simulink model "ss512"  (Simulink 8.1)
settings: Solver=ode45  StartTime=0.0  StopTime=50  FixedStep=T  RelTol=1e-3
values from neighbouring files (symbols this model uses):
  A = [0 1; 0 0]    [ss1_init.m]    (also in ss512_init.m = [0 0 1 0; ss51_init.m = [0 0 1 0)
  B = [0; 1]    [ss1_init.m]    (also in ss512_init.m = [0; 0; 0; 1]; ss51_init.m = [0; 0; 0; 1])
  C = eye(2)    [ss1_init.m]    (also in ss512_init.m = eye(n); ss51_init.m = eye(n))
  D = [0; 0]    [ss1_init.m]    (also in ss512_init.m = zeros([n 1]); ss51_init.m = zeros([n 1]))
  H = [1 0]    [ex8_init.m]    (also in ss512_init.m = [1 0 0 0])
  K1 = myacker(Phi, Gamma, z1)    [ss512_init.m]    (also in ss51_init.m)
  K2 = myacker(Phi, Gamma, z2)    [ss512_init.m]    (also in ss51_init.m)
  Lp = acker(Phi', H', p)'    [ex8_init.m]    (also in ss512_init.m = acker(Phi', H', z3)')
  Phi = [1 T; 0 1]    [ex8_init.m]
  T = 0.1    [ex8_init.m]    (also in ss1_init.m; ss512_init.m = 0.4; ss51_init.m = 0.4)
  x1 = [1; 0]    [ex8_init.m]    (also in ss1_init.m = [1; 1]; ss512_init.m = [1; 0; 0; 0]; ss51_init.m = [1; 0; 0; 0])
undefined symbols (not defined in the file or in its folder): Gamma
settings Model: Creator=jmahler  LastModifiedBy=jmahler
settings DataIOCC: SignalLoggingSaveFormat=Dataset
settings OptimizationCC: ExpressionDepthLimit=128
settings DebuggingCC: FcnCallInpInsideContextMsg=EnableAllAsError
settings GRTTargetCC: CombineOutputUpdateFcns=on  GRTInterface=off

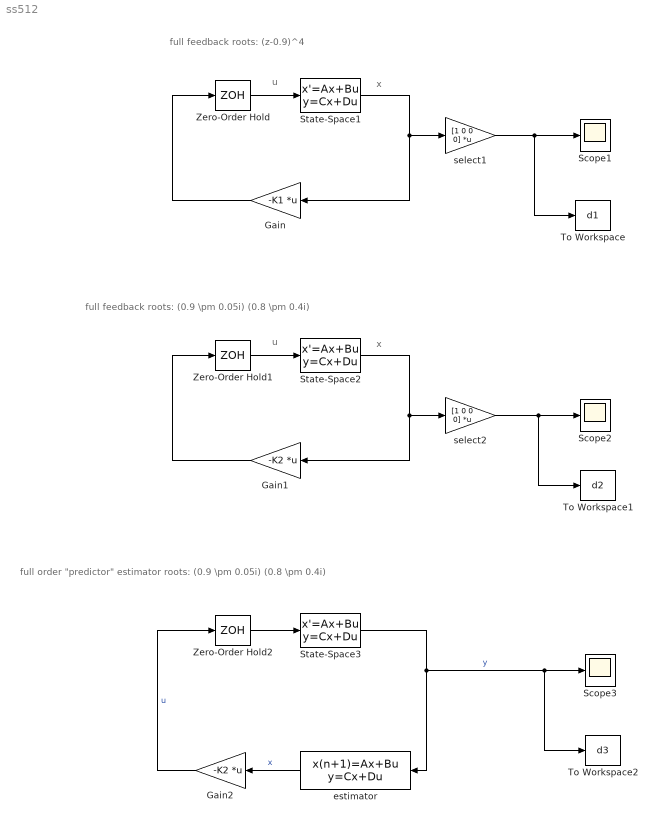
== system ss512 ==
  note: full feedback
      | roots: (z-0.9)^4
  note: u
  note: x
  note: u
  note: x
  note: full feedback
      | roots: (0.9 \pm 0.05i) (0.8 \pm 0.4i)
  note: full order "predictor" estimator
      | roots: (0.9 \pm 0.05i) (0.8 \pm 0.4i)
  Gain : Gain  Gain=-K1  Multiplication=Matrix(K*u)
  Gain1 : Gain  Gain=-K2  Multiplication=Matrix(K*u)
  Gain2 : Gain  Gain=-K2  Multiplication=Matrix(K*u)
  Scope1 : Scope
  Scope2 : Scope
  Scope3 : Scope
      settings: SaveName=ScopeData2
  State-Space1 : StateSpace  A=A  B=B  C=C  D=D  X0=x1
  State-Space2 : StateSpace  A=A  B=B  C=C  D=D  X0=x1
  State-Space3 : StateSpace  A=A  B=B  C=H  D=[0]  X0=x1
  To Workspace : ToWorkspace  VariableName=d1  SampleTime=-1  SaveFormat=Timeseries
  To Workspace1 : ToWorkspace  VariableName=d2  SampleTime=-1  SaveFormat=Timeseries
  To Workspace2 : ToWorkspace  VariableName=d3  SampleTime=-1  SaveFormat=Timeseries
  Zero-Order Hold : ZeroOrderHold  SampleTime=T
  Zero-Order Hold1 : ZeroOrderHold  SampleTime=T
  Zero-Order Hold2 : ZeroOrderHold  SampleTime=T
  estimator : DiscreteStateSpace  A=(Phi - Gamma*K2 - Lp*H)  B=Lp  C=eye(4)  D=[0; 0; 0; 0]  X0=x1  SampleTime=T
  select1 : Gain  Gain=[1 0 0 0]  Multiplication=Matrix(K*u)
  select2 : Gain  Gain=[1 0 0 0]  Multiplication=Matrix(K*u)
  wires:
  Gain/1 -> Zero-Order Hold/1
  Zero-Order Hold/1 -> State-Space1/1
  State-Space1/1 -> select1/1, Gain/1
  Gain1/1 -> Zero-Order Hold1/1
  Zero-Order Hold1/1 -> State-Space2/1
  State-Space2/1 -> select2/1, Gain1/1
  select1/1 -> To Workspace/1, Scope1/1
  select2/1 -> To Workspace1/1, Scope2/1
  Zero-Order Hold2/1 -> State-Space3/1
  Gain2/1 -> Zero-Order Hold2/1  "u"
  estimator/1 -> Gain2/1  "x"
  State-Space3/1 -> To Workspace2/1, Scope3/1, estimator/1  "y"
